simulink model "manoeuvreSV"  (Simulink 7.5)
settings: Solver=ode45  StartTime=0.0  StopTime=10.0  RelTol=1e-3
settings Model: Creator=paris  LastModifiedBy=paris

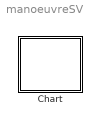
== system manoeuvreSV ==
  Chart : Stateflow chart  TreatAsAtomicUnit=on

== stateflow chart Chart ==
  state MANOEUVRESORTIEDEVOIE
    state SORTIE1 DE VOIE GAUCHE (CENTRE)
      state HORS DE VOIE
        state Recentration
        state Excentration
        MANOEUVRESORTIEDEVOIE.SORTIE1.HORS.Excentration -> MANOEUVRESORTIEDEVOIE.SORTIE1.HORS.Recentration : [ml.progression_SV==-1]
      state DANS VOIE
      MANOEUVRESORTIEDEVOIE.SORTIE1.HORS.Recentration -> MANOEUVRESORTIEDEVOIE.SORTIE1.DANS VOIE : [ml.etat_SV==0]
    state IMMINENTE
    state SORTIE DE VOIE DROITE (ACCOTEMENT)
      state HORS DE VOIE
        state Recentration
        state Excentration
        MANOEUVRESORTIEDEVOIE.SORTIE.HORS.Excentration -> MANOEUVRESORTIEDEVOIE.SORTIE.HORS.Recentration : [ml.progression_SV==-1]
      state IMMINENTE
      state DANS VOIE
      MANOEUVRESORTIEDEVOIE.SORTIE.HORS.Recentration -> MANOEUVRESORTIEDEVOIE.SORTIE.DANS VOIE : [ml.etat_SV==0]
      (default) -> MANOEUVRESORTIEDEVOIE.SORTIE.IMMINENTE : [ml.tlcCalcule<=1]
      MANOEUVRESORTIEDEVOIE.SORTIE.IMMINENTE -> MANOEUVRESORTIEDEVOIE.SORTIE.HORS.Excentration : [ml.progression_SV==1]
    (default) -> (junction 16) [order 3] : [ml.lateralisation_SV==-1]
    (default) -> (junction 17) [order 2] : [ml.lateralisation_SV==1]
    (default) -> MANOEUVRESORTIEDEVOIE.IMMINENTE [order 1] : [ml.tlcCalcule<=1]
    MANOEUVRESORTIEDEVOIE.IMMINENTE -> MANOEUVRESORTIEDEVOIE.SORTIE1.HORS.Excentration : [ml.progression_SV==1]
